simulink model "nonlinear_model"  (R2021a)
settings: Solver=ode4  StartTime=0.0  StopTime=200  FixedStep=0.001  RelTol=1e-3
settings Model: Creator=phy31  LastModifiedBy=phy31
settings SolverCC: ODENIntegrationMethod=ode14x
settings DataIOCC: SaveState=on

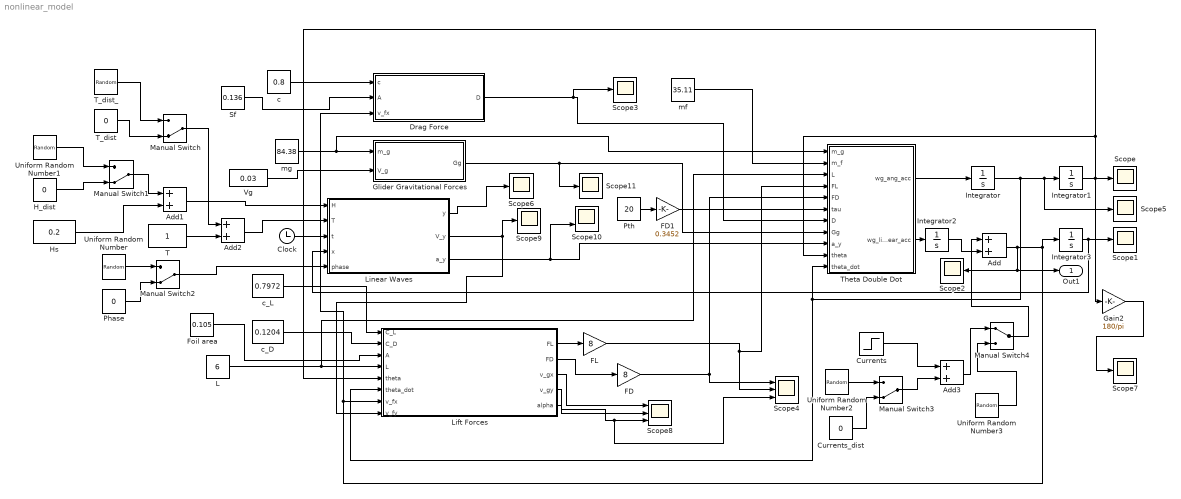
== system nonlinear_model ==
  Add{,1..3} (4 alike) : Sum
  Clock : Clock
  Currents : Step  Time=25  After=0  SampleTime=0
  Currents_dist : Constant  Value=0
  Drag Force : MATLAB Function  TreatAsAtomicUnit=on
  FD : Gain  Gain=8
  FD1 : Gain  Gain=0.3452
  FL : Gain  Gain=8
  Foil area : Constant  Value=0.105
  Gain2 : Gain  Gain=180/pi
  Glider Gravitational Forces : MATLAB Function  TreatAsAtomicUnit=on
  H_dist : Constant  Value=0
  Hs : Constant  Value=0.2
  Integrator : Integrator
  Integrator1 : Integrator  LimitOutput=on  UpperSaturationLimit=pi/2  LowerSaturationLimit=-pi/2
  Integrator2 : Integrator
  Integrator3 : Integrator
  L : Constant  Value=6
  Lift Forces : MATLAB Function  TreatAsAtomicUnit=on
  Linear Waves : MATLAB Function  TreatAsAtomicUnit=on
  Manual Switch{,1..3} (4 alike) : ManualSwitch  CurrentSetting=0
  Manual Switch4 : ManualSwitch
  Phase : Constant  Value=0
  Pth : Constant  Value=20
  Scope{,1..3,5..7,9,11} (9 alike) : Scope
  Scope10 : Scope  NumInputPorts=2
  Scope4 : Scope  NumInputPorts=3
  Scope8 : Scope  NumInputPorts=3
  Sf : Constant  Value=0.136
  T : Constant
  T_dist : Constant  Value=0
  T_dist_ : UniformRandomNumber  Minimum=-1.8  Maximum=1.8  SampleTime=1
  Theta Double Dot : MATLAB Function  TreatAsAtomicUnit=on
  Uniform Random Number : UniformRandomNumber  Minimum=-pi  Maximum=pi  SampleTime=1
  Uniform Random Number1 : UniformRandomNumber  Minimum=-0.5  Maximum=0.5  SampleTime=1
  Uniform Random Number2 : UniformRandomNumber  Minimum=-0.5  Maximum=0.5  SampleTime=0.1
  Uniform Random Number3 : UniformRandomNumber  Minimum=-0.5  Maximum=0.5  SampleTime=1
  Vg : Constant  Value=0.03
  c : Constant  Value=0.8
  c_D : Constant  Value=0.1204
  c_L : Constant  Value=0.7972
  mf : Constant  Value=35.11
  mg : Constant  Value=84.38
  Out1 : Outport
  wires:
  Sf/1 -> Drag Force/2(A)
  c/1 -> Drag Force/1(c)
  mg/1 -> Theta Double Dot/1(m_g), Glider Gravitational Forces/1(m_g)
  Vg/1 -> Glider Gravitational Forces/2(V_g)
  Clock/1 -> Linear Waves/3(t)
  c_L/1 -> Lift Forces/1(C_L)
  Foil area/1 -> Lift Forces/3(A)
  L/1 -> Theta Double Dot/3(L), Lift Forces/4(L)
  mf/1 -> Theta Double Dot/2(m_f)
  Lift Forces/1(FL) -> FL/1
  Pth/1 -> FD1/1
  Drag Force/1(D) -> Scope3/1, Theta Double Dot/7(D)
  Glider Gravitational Forces/1(Gg) -> Scope11/1, Theta Double Dot/8(Gg)
  Linear Waves/3(a_y) -> Scope10/2, Theta Double Dot/9(a_y)
  Theta Double Dot/1(wg_ang_acc) -> Integrator/1
  Integrator/1 -> Theta Double Dot/11(theta_dot), Lift Forces/6(theta_dot), Scope5/1, Integrator1/1
  Add/1 -> Scope2/1, Out1/1, Drag Force/3(v_fx), Lift Forces/7(v_fx), Integrator3/1
  Integrator1/1 -> Gain2/1, Lift Forces/5(theta), Theta Double Dot/10(theta), Scope/1
  FD/1 -> Scope4/1, Theta Double Dot/5(FD)
  Lift Forces/2(FD) -> FD/1
  Linear Waves/2(V_y) -> Lift Forces/8(v_fy), Scope9/1
  FL/1 -> Scope4/2, Theta Double Dot/4(FL)
  Linear Waves/1(y) -> Scope6/1
  Gain2/1 -> Scope7/1
  c_D/1 -> Lift Forces/2(C_D)
  Integrator3/1 -> Linear Waves/4(x), Scope1/1
  Lift Forces/3(v_gx) -> Scope8/1
  Lift Forces/4(v_gy) -> Scope8/2
  Lift Forces/5(alpha) -> Scope4/3, Scope8/3
  Theta Double Dot/2(wg_linear_acc) -> Integrator2/1
  Integrator2/1 -> Add/2
  Hs/1 -> Add1/2
  Add1/1 -> Linear Waves/1(H)
  T/1 -> Add2/2
  Add2/1 -> Linear Waves/2(T)
  T_dist_/1 -> Manual Switch/1
  Manual Switch/1 -> Add2/1
  T_dist/1 -> Manual Switch/2
  Manual Switch1/1 -> Add1/1
  Uniform Random Number1/1 -> Manual Switch1/1
  H_dist/1 -> Manual Switch1/2
  Manual Switch2/1 -> Linear Waves/5(phase)
  Uniform Random Number/1 -> Manual Switch2/1
  Phase/1 -> Manual Switch2/2
  Manual Switch3/1 -> Add3/2
  Currents/1 -> Add3/1
  Currents_dist/1 -> Manual Switch3/2
  Uniform Random Number2/1 -> Manual Switch3/1
  FD1/1 -> Theta Double Dot/6(tau)
  Add3/1 -> Manual Switch4/1
  Manual Switch4/1 -> Add/1
  Uniform Random Number3/1 -> Manual Switch4/2

== matlab function nonlinear_model/Lift Forces ==
  data: C_L input; FL output; C_D input; FD output; A input; L input; theta input; theta_dot input; v_fx input; v_fy input; v_gx output; v_gy output; alpha output
function [FL,FD,v_gx, v_gy, alpha] = fcn(C_L,C_D,A,L,theta,theta_dot,v_fx,v_fy)
v_gx = v_fx + L*theta_dot*cos(theta);
v_gy = v_fy + L*theta_dot*sin(theta);
v_g = sqrt(v_gx^2 + v_gy^2);
FL_c = 0.5*1015*A*C_L*(v_g)^2;
FD_c = 0.5*1015*A*C_D*(v_g)^2;

alpha = atan2(abs(v_gy), abs(v_gx));
%alpha2 = atan2((v_gy),(v_gx));

if alpha > pi/8
    alpha = pi/8;
end

FL = FL_c*sin(alpha) - FD_c*cos(alpha);
FD = -FL_c*cos(alpha) - FD_c*sin(alpha);

if v_gy < 0
    FD = FD * -1;
end

== matlab function nonlinear_model/Linear Waves ==
  data: H input; y output; T input; V_y output; t input; x input; phase input; a_y output
function [y,V_y,a_y] = fcn(H,T,t,x,phase)
lambda = 9.81*T^2 / (2*pi);
omega = 2*pi / T;
k = 2*pi / lambda;
theta = k*x-omega*t+phase;
y = (H/2)*sin(theta);
V_y = (-1)*omega*(H/2)*cos(theta);
a_y = (-1)*(omega^2)*(H/2)*sin(theta);

== matlab function nonlinear_model/Drag Force ==
  data: c input; D output; A input; v_fx input
function D  = fcn(c,A,v_fx)
D = 0.5*1015*A*c*abs(v_fx)*v_fx;

== matlab function nonlinear_model/Glider Gravitational Forces ==
  data: m_g input; Gg output; V_g input
function Gg  = fcn(m_g, V_g)
Gg = m_g*9.81 - 1015*9.81*V_g;

== matlab function nonlinear_model/Theta Double Dot ==
  data: m_g input; wg_ang_acc output; m_f input; L input; FL input; FD input; tau input; D input; Gg input; a_y input; theta input; theta_dot input; wg_linear_acc output
function [wg_ang_acc,wg_linear_acc] = fcn(m_g, m_f, L, FL, FD, tau, D, Gg, a_y, theta, theta_dot)
c1 = -1/(m_g*L*(m_f+m_g*(sin(theta)^2)));
c2 = m_g*cos(theta)*(FL+tau-D+m_g*L*((theta_dot)^2)*sin(theta));
c3 = (m_f+m_g)*((FL+tau)*cos(theta) - (Gg+FD)*sin(theta) - m_g*a_y*sin(theta));

wg_ang_acc = c1*(c2-c3);

c4 = 1/(m_f+m_g*(sin(theta)^2));
c5 = (FL+tau)*(sin(theta)^2) + (Gg+FD+m_g*a_y)*sin(theta)*cos(theta) + m_g*L*(theta_dot^2)*sin(theta) - D;

wg_linear_acc = c4*c5;
